simulink model "chap11_4sim"  (R2023b)
settings: Solver=ode45  StartTime=0.0  StopTime=5  RelTol=1e-3
values from neighbouring files (symbols this model uses):
  b = 1    [chap11_4int.m]    (also in chap11_6int.m = 0.5)
  bc = 30.0    (= 30)    [chap11_4int.m]
  bc1 = bc/Gain    (= 0.454545454545)    [chap11_4int.m]
  Ce = 0.001    [chap11_4int.m]
  Fc = 0.28    [chap11_1plant.m]    (also in chap11_4int.m = 100)
  Fc1 = Fc/Gain    (= 1.51515151515)    [chap11_4int.m]
  J = 1.0    (= 1)    [chap11_1plant.m]    (also in chap11_4int.m = 2; chap11_6int.m = 2)
  kd = 6    [chap11_4int.m]    (also in chap11_6int.m)
  kdd = 1.5    [chap11_4int.m]
  ki = 0.001    [chap11_4int.m]
  kii = 0.1    [chap11_4int.m]
  km = 1.0    (= 1)    [chap11_4int.m]
  kpp = 150    [chap11_4int.m]
  ku = 11    [chap11_4int.m]
  kv = 2    [chap11_4int.m]    (also in chap11_6int.m)
  L = 0.001    [chap11_4int.m]
  R = 1    [chap11_4int.m]
undefined symbols (not defined in the file or in its folder): sgn
settings Model: Creator=CorgiQvm  LastModifiedBy=CorgiQvm
settings DataIOCC: SaveFormat=Array  ReturnWorkspaceOutputs=off
settings ModelReferenceCC: PropagateSignalLabelsOutOfModel=off

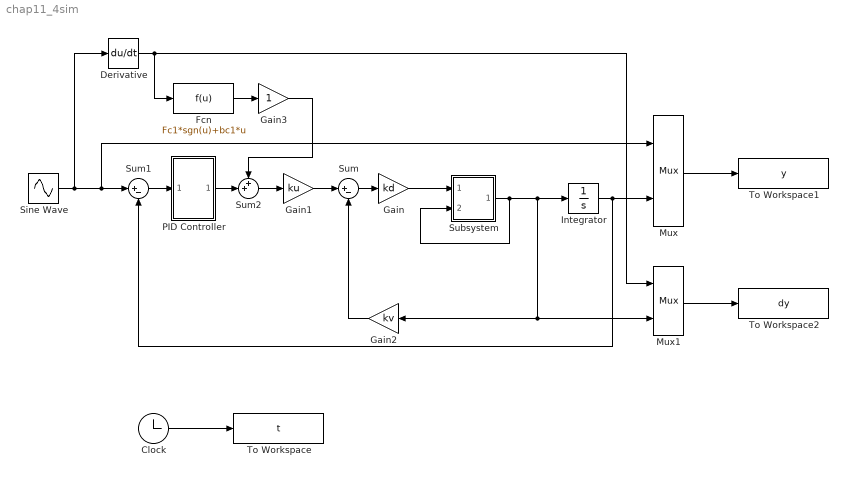
== system chap11_4sim ==
  Clock : Clock
  Derivative : Derivative
  Fcn : Fcn  Expr=Fc1*sgn(u)+bc1*u
  Gain : Gain  Gain=kd  SaturateOnIntegerOverflow=on  OutDataTypeStr=Inherit: Same as input  ParamDataTypeStr=Inherit: Same as input
  Gain1 : Gain  Gain=ku  SaturateOnIntegerOverflow=on  OutDataTypeStr=Inherit: Same as input  ParamDataTypeStr=Inherit: Same as input
  Gain2 : Gain  Gain=kv  SaturateOnIntegerOverflow=on  OutDataTypeStr=Inherit: Same as input  ParamDataTypeStr=Inherit: Same as input
  Gain3 : Gain  SaturateOnIntegerOverflow=on  OutDataTypeStr=Inherit: Same as input  ParamDataTypeStr=Inherit: Same as input
  Integrator : Integrator
  Mux : Mux  Inputs=2
  Mux1 : Mux  Inputs=2
  PID Controller : Subsystem  mask{P=kpp, I=kii, D=kdd}
      mask prompts: P "Proportional"; I "Integral"; D "Derivative"
      mask DialogControl ParameterGroupVar Prompt: 参数
      mask Display: disp('PID')
  Sine Wave : Sin  SampleTime=0
  Subsystem : Subsystem
  Sum : Sum  Inputs=|+-  InputSameDT=on  SaturateOnIntegerOverflow=on  OutDataTypeStr=Inherit: Same as first input
  Sum1 : Sum  Inputs=|+-  InputSameDT=on  SaturateOnIntegerOverflow=on  OutDataTypeStr=Inherit: Same as first input
  Sum2 : Sum  Inputs=++|  InputSameDT=on  SaturateOnIntegerOverflow=on  OutDataTypeStr=Inherit: Same as first input
  To Workspace : ToWorkspace  VariableName=t  SampleTime=-1
  To Workspace1 : ToWorkspace  VariableName=y  SampleTime=-1
  To Workspace2 : ToWorkspace  VariableName=dy  SampleTime=-1
  wires:
  Sine Wave/1 -> Derivative/1, Mux/1, Sum1/1
  Sum1/1 -> PID Controller/1(In_1)
  Gain1/1 -> Sum/1
  Sum/1 -> Gain/1
  Gain/1 -> Subsystem/1(In1)
  Subsystem/1(Out1) -> Subsystem/2(In2), Gain2/1, Mux1/2, Integrator/1
  Gain2/1 -> Sum/2
  Clock/1 -> To Workspace/1
  Derivative/1 -> Fcn/1, Mux1/1
  Mux1/1 -> To Workspace2/1
  Mux/1 -> To Workspace1/1
  Integrator/1 -> Mux/2, Sum1/2
  Sum2/1 -> Gain1/1
  PID Controller/1(Out1) -> Sum2/2
  Fcn/1 -> Gain3/1
  Gain3/1 -> Sum2/1

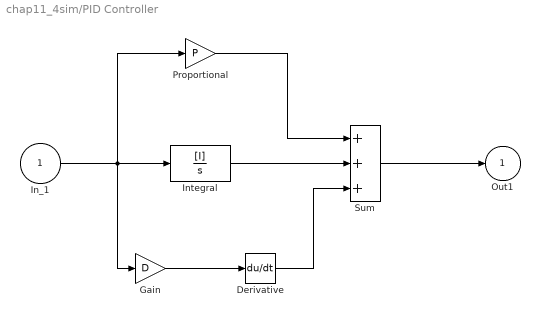
== system chap11_4sim/PID Controller ==
  In_1 : Inport
  Derivative : Derivative
  Gain : Gain  Gain=D  SaturateOnIntegerOverflow=on  OutDataTypeStr=Inherit: Same as input  ParamDataTypeStr=Inherit: Same as input
  Integral : TransferFcn  Numerator=[I]  Denominator=[1 0]
  Proportional : Gain  Gain=P  SaturateOnIntegerOverflow=on  OutDataTypeStr=Inherit: Same as input  ParamDataTypeStr=Inherit: Same as input
  Sum : Sum  Inputs=+++  InputSameDT=on  SaturateOnIntegerOverflow=on  OutDataTypeStr=Inherit: Same as first input
  Out1 : Outport
  wires:
  Derivative/1 -> Sum/3
  Proportional/1 -> Sum/1
  Sum/1 -> Out1/1
  Integral/1 -> Sum/2
  In_1/1 -> Gain/1, Proportional/1, Integral/1
  Gain/1 -> Derivative/1

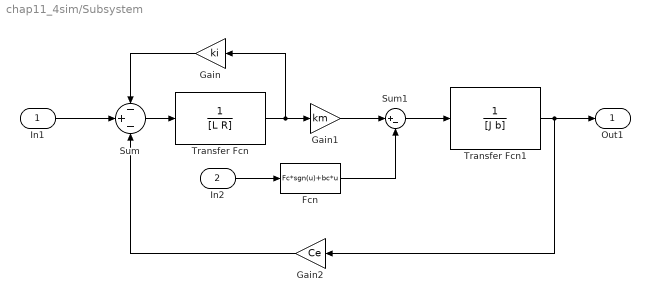
== system chap11_4sim/Subsystem ==
  In1 : Inport
  In2 : Inport  Port=2
  Fcn : Fcn  Expr=Fc*sgn(u)+bc*u
  Gain : Gain  Gain=ki  SaturateOnIntegerOverflow=on  OutDataTypeStr=Inherit: Same as input  ParamDataTypeStr=Inherit: Same as input
  Gain1 : Gain  Gain=km  SaturateOnIntegerOverflow=on  OutDataTypeStr=Inherit: Same as input  ParamDataTypeStr=Inherit: Same as input
  Gain2 : Gain  Gain=Ce  SaturateOnIntegerOverflow=on  OutDataTypeStr=Inherit: Same as input  ParamDataTypeStr=Inherit: Same as input
  Sum : Sum  Inputs=-+-  InputSameDT=on  OutDataTypeStr=Inherit: Same as first input
  Sum1 : Sum  Inputs=|+-  OutDataTypeStr=Inherit: Same as first input
  Transfer Fcn : TransferFcn  Denominator=[L R]
  Transfer Fcn1 : TransferFcn  Denominator=[J b]
  Out1 : Outport
  wires:
  Sum/1 -> Transfer Fcn/1
  Transfer Fcn/1 -> Gain1/1, Gain/1
  Transfer Fcn1/1 -> Out1/1, Gain2/1
  In2/1 -> Fcn/1
  Sum1/1 -> Transfer Fcn1/1
  Gain1/1 -> Sum1/1
  Fcn/1 -> Sum1/2
  In1/1 -> Sum/2
  Gain/1 -> Sum/1
  Gain2/1 -> Sum/3
